simulink model "Wall_Model_Version_1_8_2016a"  (R2016a)
settings: Solver=ode3  StartTime=0.0  StopTime=inf  FixedStep=Ts  RelTol=1e-3
InitFcn:
  | clc;
  | clear all;
  | close all;
  | addpath('D:\Aravind_A0164966M_EE5003\Matlab files\3r2c model')
  | Ts=1
  | Duration=36000;
  | %% Coefficients of Rs and Cs
  | 
  | %% Front Wall
  | l1 = 7.37;
  | b1 = 2.63;
  | y1 = 0.5;
  | x1 = 0.33;
  | y2 = 0.5;
  | x2 = 0.33;
  | x3 = 0.33;
  | 
  | %% Left Wall
  | l2 = 10.11;
  | b2 = 2.63;
  | y3 = 0.5;
  | x4 = 0.33;
  | y4 = 0.5;
  | x5 = 0.33;
  | x6 = 0.33;
  | 
  | %% Left Wall Glass
  | x4_g = 0.5;
  | x5_g = 0.5;
  | y3_g = 1;
  | 
  | %% Right Wall
  | l3 = 7.37;
  | b3 = 2.63;
  | y5 = 0.5;
  | x7 = 0.33;
  | y6 = 0.5;
  | x8 = 0.33;
  | x9 = 0.33;
  | 
  | %% Back Wall
  | l4 = 10.11;
  | b4 = 2.63;
  | y7 = 1;
  | x10 = 0.5;
  | %y8 = 0.5;
  | x11 = 0.5;
  | %x12= 0.33;
  | 
  | %% Roof
  | l5 = 10.11;
  | b5 = 7.37;
  | y9 = 0.5;
  | x13 = 0.33;
  | y10 = 0.5;
  | x14 = 0.33;
  | x15 = 0.33;
  | 
  | %% Floor
  | l6 = 10.11;
  | b6 = 7.37;
  | y11 = 0.5;
  | x16 = 0.33;
  | y12 = 0.5;
  | x17 = 0.33;
  | x18 = 0.33;
  | 
  | %%Areas
  | A1 = l1 * b1;
  | A2 = l2 * b2;
  | A3 = l3 * b3;
  | A4 = l4 * b4;
  | A5 = l5 * b5;
  | A6 = l6 * b6;
  | 
  | %% Initial Temperatures at the surfaces
  | T1_initial_front=301;
  | T2_initial_front=300;
  | 
  | T1_initial_left=301;
  | T2_initial_left=300;
  | 
  | T1_initial_right=301;
  | T2_initial_right=300;
  | 
  | T1_initial_back=301;
  | T2_initial_back=300;
  | 
  | T1_initial_roof=301;
  | T2_initial_roof=300;
  | 
  | T1_initial_floor=301;
  | T2_initial_floor=300;
  | 
  | %ri = 0.1300; % m2 K/W resistance of inner surface of brick wall
  | %rso = 0.04; % m2 K/W resistance of outer surface of the wall
  | 
  | ri = 0;
  | rso = 0;
  | %% Density of Building materials in the room
  | p_conc    = 2400; % kg/m3 density of concrete
  | p_pstr     = 850; % kg/m3 density of plastering
  | p_gb       = 1100; % kg/m3 density of gypsum board
  | p_glass    = 2530; % kg/m3 density of glass
  | p_swood  = 550;   % kg/m3 density of soft-wood
  | 
  | %% Thermal heat capacity of the building materials in the room
  | c_conc    = 840;  % J/kg K heat capacity of concrete
  | c_pstr     = 1000;  %J/kg K heat capacity of plastering
  | c_gb       = 700; % J/kg K heat capacity of gypsum board
  | c_glass    = 840;  % J/kg K heat capacity of glass
  | c_swood  = 1700; % J/kg K heat capacity of soft-wood
  | 
  | %% Thermal conductivity(lamda) of building materials in the room
  | l_conc    = 0.8;  % W/m K Thermal conductivity of concrete
  | l_pstr     = 0.013;  % W/m K Thermal conductivity of plastering
  | l_gb       = 0.35; % W/m K Thermal conductivity of gypsum board
  | l_glass    = 0.8;  % W/m K Thermal conductivity of glass
  | l_swood  = 0.08; % W/m K Thermal conductivity of soft-wood
  | 
  | %% Standard thickness of materials used
  | d_conc = 0.01;  % m Thickness of concrete BCA standard
  | d_pstr = 0.005; % m Thickness of plastering BCA standard
  | d_glass = 0.015; % m Thickness of glass wall widely used
  | d_swood = 0.01; % m Thickness of softwood on the right wall
  | d_gb = 0.015; % m Thickness of gypsum board
  | 
  | %% Resistance and Capacitance of front Wall
  | Rth1 =( ri + rso + (d_conc/l_conc) + (d_pstr/l_pstr))/(A1); % Thermal resistance
  | Cth1 = A1*(d_conc*p_conc*c_conc + d_pstr*p_pstr*c_pstr) ; % Thermal Capacitance
  | 
  | %% Resistance and Capacitance of left Wall concrete
  | A_conc = A2 * 0.5; % Half of the wall on the left is  glass wall
  | Rth2 =( ri + rso + (d_conc/l_conc) + (d_pstr/l_pstr))/(A_conc); % Thermal resistance
  | Cth2 = A_conc*(d_conc*p_conc*c_conc + d_pstr*p_pstr*c_pstr); % Thermal Capacitance
  | 
  | %% Resistance and Capacitance of left Wall glass
  | A_glass = A2 * 0.5; % Half of the wall on the left is  glass wall
  | Rth2_g =(d_glass/l_glass) /(A_glass); % Thermal resistance
  | Cth2_g = A_glass*(d_glass*p_glass*c_glass ); % Thermal Capacitance
  | 
  | %% Resistance and Capacitance of right Wall
  | Rth3 = ( ri + rso+ (d_conc/l_conc) + (d_swood/l_swood))/(A3);% Thermal resistance
  | Cth3 = A3*(d_swood*p_swood*c_swood + d_conc*p_conc*c_conc ); % Thermal Capacitance
  | 
  | %% Resistance and Capacitance of back Wall
  | Rth4 =(d_glass/l_glass) /(A4); % Thermal resistance
  | Cth4 = A4*(d_glass*p_glass*c_glass ); % Thermal Capacitance
  | 
  | %% Resistance and Capacitance of roof Wall
  | Rth5 = (d_gb/l_gb)/(A5);% Thermal resistance
  | Cth5 = A5*(d_gb*p_gb*c_gb ); % Thermal Capacitance
  | 
  | %% Resistance and Capacitance of floor Wall
  | Rth6 = (d_gb/l_gb)/(A6);% Thermal resistance
  | Cth6 = A6*(d_gb*p_gb*c_gb ); % Thermal Capacitance
  | 
  | %% Volume and mass of room
  | density_of_air = 1.184; % kg/m3 at 25 deg. K
  | volume = l1*l2*b1; % m3
  | mass = volume * density_of_air ;% kg
  | specific_heat = 1.005; % J/kg deg.K
  | tic;
libraries: powerlib x70, simulink x1
settings Model: Creator=elekkr  LastModifiedBy=e0154145
settings DataIOCC: LimitDataPoints=on  SaveFormat=Array
settings DebuggingCC: UnconnectedInputMsg=none  UnconnectedOutputMsg=none  UnconnectedLineMsg=none
settings HardwareCC: ProdBitPerPointer=32  ProdLargestAtomicFloat=None  ProdIntDivRoundTo=Undefined  ProdEndianess=Unspecified  ProdWordSize=32  ProdHWDeviceType=32-bit Generic
settings ModelReferenceCC: PropagateSignalLabelsOutOfModel=off
settings SimscapeCC: SimscapeNormalizeSystem=off

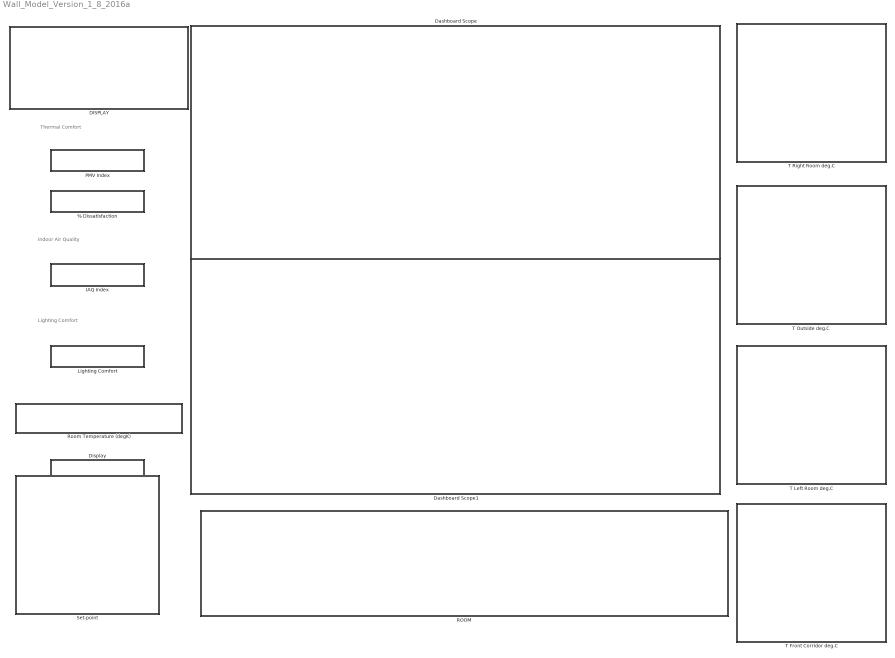
== system Wall_Model_Version_1_8_2016a ==
  note: Thermal Comfort
  note: Indoor Air Quality
  note: Lighting Comfort
  % Dissatisfaction : Subsystem  Description=Replaced Block  mask(Replaced Block){}
      mask help: This block has been replaced with an empty subsystem because it used functionality that is unavailable in Simulink R2016a.
      mask Display: fprintf('Replaced: %s\n','Dashboard Widget')
  DISPLAY : Subsystem  mask(GBIC - Simulation Speed){}
      settings: AttributesFormatString=141.41
      mask Display: fprintf('Simulation_Time_Elapsed=3536.00 seconds\nPhysical_Time_Elapsed=70.38 seconds\nSimulation_Speed=50.24 times')
  Dashboard Scope : Subsystem  DialogController=hmiCreateDDGDialog  IsWebBlock=on  mask(MWDashboardBlock){webBlockId=3fff6f15-1f4d-4564-ab32-a1e668a3884d, webBlockType=sdiscope, ShowInitialText=on, HMISrcModelName=Wall_Model_Version_1_8_2016a}
      mask prompts: webBlockId "WebBlock Id"; webBlockType "WebBlock Type"; HMISrcModelName "Source Model"
      mask help: SimulinkHMI:dialogs:HMIScopeDialogDesc
      mask Help: helpview([docroot '/mapfiles/simulink.map'], 'hmi_scope')
      mask Display:
      | if strcmp(get_param(bdroot(gcb),'BlockDiagramType'), 'library')
      |     image([(matlabroot) '/toolbox/simulink/hmi/icons/DashboardScope.png']);
      | end
  Dashboard Scope1 : Subsystem  DialogController=hmiCreateDDGDialog  IsWebBlock=on  mask(MWDashboardBlock){webBlockId=a7778c0b-7014-479c-88b7-c1742b1b2716, webBlockType=sdiscope, ShowInitialText=on, HMISrcModelName=Wall_Model_Version_1_8_2016a}
      mask prompts: webBlockId "WebBlock Id"; webBlockType "WebBlock Type"; HMISrcModelName "Source Model"
      mask help: SimulinkHMI:dialogs:HMIScopeDialogDesc
      mask Help: helpview([docroot '/mapfiles/simulink.map'], 'hmi_scope')
      mask Display:
      | if strcmp(get_param(bdroot(gcb),'BlockDiagramType'), 'library')
      |     image([(matlabroot) '/toolbox/simulink/hmi/icons/DashboardScope.png']);
      | end
  Display : Subsystem  Description=Replaced Block  mask(Replaced Block){}
      mask help: This block has been replaced with an empty subsystem because it used functionality that is unavailable in Simulink R2016a.
      mask Display: fprintf('Replaced: %s\n','Dashboard Widget')
  IAQ Index : Subsystem  Description=Replaced Block  mask(Replaced Block){}
      mask help: This block has been replaced with an empty subsystem because it used functionality that is unavailable in Simulink R2016a.
      mask Display: fprintf('Replaced: %s\n','Dashboard Widget')
  Lighting Comfort : Subsystem  Description=Replaced Block  mask(Replaced Block){}
      mask help: This block has been replaced with an empty subsystem because it used functionality that is unavailable in Simulink R2016a.
      mask Display: fprintf('Replaced: %s\n','Dashboard Widget')
  PMV Index : Subsystem  Description=Replaced Block  mask(Replaced Block){}
      mask help: This block has been replaced with an empty subsystem because it used functionality that is unavailable in Simulink R2016a.
      mask Display: fprintf('Replaced: %s\n','Dashboard Widget')
  ROOM : Subsystem
  Room Temperature (degK) : Subsystem  DialogController=hmiCreateDDGDialog  IsWebBlock=on  mask(MWDashboardBlock){webBlockId=20cf081a-ecf9-409a-b722-1806c1b228f7, webBlockType=lineargauge, ShowInLibBrowser=on, ShowInitialText=on, HMISrcModelName=Wall_Model_Version_1_8_2016a}
      mask prompts: webBlockId "WebBlock Id"; webBlockType "WebBlock Type"; HMISrcModelName "Source Model"
      mask help: SimulinkHMI:dialogs:LinearGaugeDialogDesc
      mask Help: helpview([docroot '/mapfiles/simulink.map'], 'hmi_linear_gauge')
      mask Display:
      | if strcmp(get_param(bdroot(gcb),'BlockDiagramType'), 'library')
      |     image([(matlabroot) '/toolbox/simulink/hmi/icons/LinearGauge.png']);
      | end
  Set-point : Subsystem  DialogController=hmiCreateDDGDialog  IsWebBlock=on  mask(MWDashboardBlock){webBlockId=ec28f16f-92e5-498c-80e5-da4bfa106054, webBlockType=discreteknob, ShowInLibBrowser=on, ShowInitialText=on, HMISrcModelName=Wall_Model_Version_1_8_2016a}
      mask prompts: webBlockId "WebBlock Id"; webBlockType "WebBlock Type"; HMISrcModelName "Source Model"
      mask help: Set value to tune parameters or variables.
      mask Help: helpview([docroot '/mapfiles/simulink.map'], 'hmi_rotary_switch')
      mask Display:
      | if strcmp(get_param(bdroot(gcb),'BlockDiagramType'),'library')
      |  image([(matlabroot) '/toolbox/simulink/hmi/icons/DiscreteKnob.png'])
      | end
  T Front Corridor deg.C : Subsystem  DialogController=hmiCreateDDGDialog  IsWebBlock=on  mask(MWDashboardBlock){webBlockId=cdae9e03-d357-446c-8d97-860cc5abe23b, webBlockType=discreteknob, ShowInLibBrowser=on, ShowInitialText=on, HMISrcModelName=Wall_Model_Version_1_8_2016a}
      mask prompts: webBlockId "WebBlock Id"; webBlockType "WebBlock Type"; HMISrcModelName "Source Model"
      mask help: Set value to tune parameters or variables.
      mask Help: helpview([docroot '/mapfiles/simulink.map'], 'hmi_rotary_switch')
      mask Display:
      | if strcmp(get_param(bdroot(gcb),'BlockDiagramType'),'library')
      |  image([(matlabroot) '/toolbox/simulink/hmi/icons/DiscreteKnob.png'])
      | end
  T Left Room deg.C : Subsystem  DialogController=hmiCreateDDGDialog  IsWebBlock=on  mask(MWDashboardBlock){webBlockId=223c3754-b648-4b30-8efa-3705ba18b69c, webBlockType=discreteknob, ShowInLibBrowser=on, ShowInitialText=on, HMISrcModelName=Wall_Model_Version_1_8_2016a}
      mask prompts: webBlockId "WebBlock Id"; webBlockType "WebBlock Type"; HMISrcModelName "Source Model"
      mask help: Set value to tune parameters or variables.
      mask Help: helpview([docroot '/mapfiles/simulink.map'], 'hmi_rotary_switch')
      mask Display:
      | if strcmp(get_param(bdroot(gcb),'BlockDiagramType'),'library')
      |  image([(matlabroot) '/toolbox/simulink/hmi/icons/DiscreteKnob.png'])
      | end
  T Outside deg.C : Subsystem  DialogController=hmiCreateDDGDialog  IsWebBlock=on  mask(MWDashboardBlock){webBlockId=3d2b147f-38bc-43af-8396-33a98fe59ecc, webBlockType=discreteknob, ShowInLibBrowser=on, ShowInitialText=on, HMISrcModelName=Wall_Model_Version_1_8_2016a}
      mask prompts: webBlockId "WebBlock Id"; webBlockType "WebBlock Type"; HMISrcModelName "Source Model"
      mask help: Set value to tune parameters or variables.
      mask Help: helpview([docroot '/mapfiles/simulink.map'], 'hmi_rotary_switch')
      mask Display:
      | if strcmp(get_param(bdroot(gcb),'BlockDiagramType'),'library')
      |  image([(matlabroot) '/toolbox/simulink/hmi/icons/DiscreteKnob.png'])
      | end
  T Right Room deg.C : Subsystem  DialogController=hmiCreateDDGDialog  IsWebBlock=on  mask(MWDashboardBlock){webBlockId=eb2fffaf-f8f3-43a1-940d-0b33cab81fdd, webBlockType=discreteknob, ShowInLibBrowser=on, ShowInitialText=on, HMISrcModelName=Wall_Model_Version_1_8_2016a}
      mask prompts: webBlockId "WebBlock Id"; webBlockType "WebBlock Type"; HMISrcModelName "Source Model"
      mask help: Set value to tune parameters or variables.
      mask Help: helpview([docroot '/mapfiles/simulink.map'], 'hmi_rotary_switch')
      mask Display:
      | if strcmp(get_param(bdroot(gcb),'BlockDiagramType'),'library')
      |  image([(matlabroot) '/toolbox/simulink/hmi/icons/DiscreteKnob.png'])
      | end

== system Wall_Model_Version_1_8_2016a/% Dissatisfaction ==

== system Wall_Model_Version_1_8_2016a/DISPLAY ==
  Disp_Function : M-S-Function  FunctionName=fn_Display

== system Wall_Model_Version_1_8_2016a/Dashboard Scope ==

== system Wall_Model_Version_1_8_2016a/Dashboard Scope1 ==

== system Wall_Model_Version_1_8_2016a/Display ==

== system Wall_Model_Version_1_8_2016a/IAQ Index ==

== system Wall_Model_Version_1_8_2016a/Lighting Comfort ==

== system Wall_Model_Version_1_8_2016a/PMV Index ==

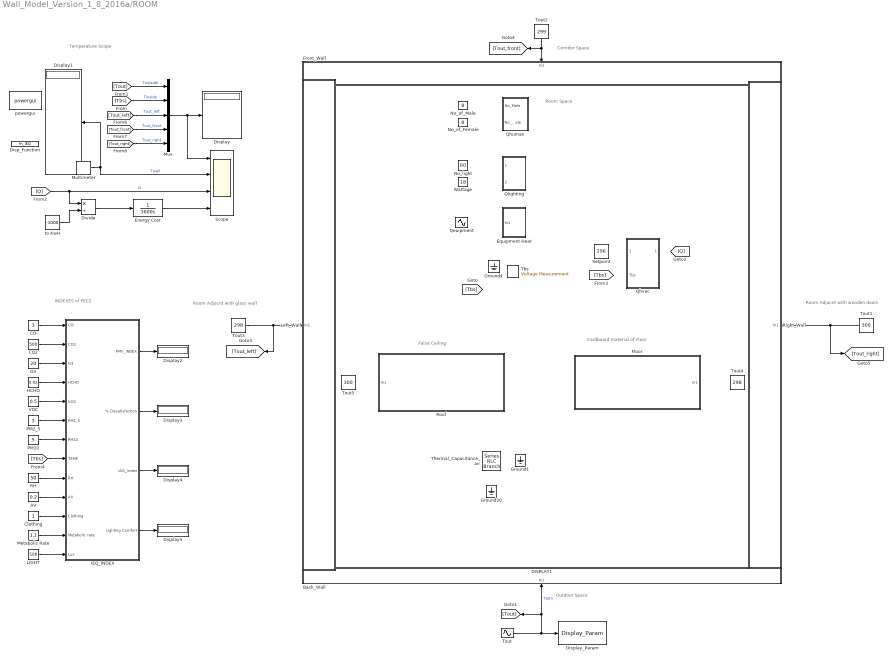
== system Wall_Model_Version_1_8_2016a/ROOM ==
  note: INDEXES of FEC2
  note: False Ceiling
  note: Cardboard material of Floor
  note: Room Adjacnt with wooden doors
  note: Corridor Space
  note: Room Adjacnt with glass wall
  note: Outdoor Space
  note: Room Space
  note: Temperature Scope
  AV : Constant  Value=0.2
  Back_Wall : Subsystem
      mask Display: fprintf('Temperature Outside= 303 deg. K\n')
  CO : Constant  Value=3
  CO2 : Constant  Value=500
  Clothing : Constant
  DISPLAY1 : Subsystem  mask(GBIC - Simulation Speed){}
      settings: AttributesFormatString=35.01
  Disp_Function : M-S-Function  FunctionName=fn_IEQ
  Display{,1..5} (6 alike) : Display
  Display_Param : M-S-Function  FunctionName=Display_Param
  Divide : Product  Inputs=*/
  Energy Cost : TransferFcn  Denominator=[3600 0]
  Equipment Heat : Subsystem
  Floor : Subsystem
      mask Display: fprintf('Temperature \n Below= \n298 deg. K\n')
  Front_Wall : Subsystem
      mask Display: fprintf('Temperature Corridor= 299 deg. K\n')
  Ground1 : powerlib/Elements/Ground  LConnTagsString=a
  Ground20 : powerlib/Elements/Ground  LConnTagsString=a
  Ground4 : powerlib/Elements/Ground  LConnTagsString=a
  HCHO : Constant  Value=0.02
  IEQ_INDEX : Subsystem
  LIGHT : Constant  Value=500
  Left_Wall : Subsystem
      mask Display: fprintf('Temperature \n Left Room= \n298 deg. K\n')
  Metabolic Rate : Constant  Value=1.1
  Multimeter : powerlib/Measurements/Multimeter  PhasorSimulation=off  OutputType=Complex  sel=1  L=12  Gain=0  yselected={}  PSBOutputType=1  PSBequivalent=0  AxesSetting=[0,0.1,-100,100]  Display=0  SavedBlockNames=-11
  Mux : Mux  Inputs=5
  No_light : Constant  Value=60
  No_of_Female : Constant  Value=8
  No_of_Male : Constant  Value=8
  O3 : Constant  Value=20
  PM10 : Constant  Value=5
  PM2_5 : Constant  Value=3
  Qeuipment : Sin  Amplitude=200  Bias=3200  Frequency=2*pi/(12*3600)  SampleTime=0
  Qhuman : Subsystem
  Qhvac : Subsystem
  Qlighting : Subsystem
  RH : Constant  Value=50
  Right_Wall : Subsystem
      mask Display: fprintf('Temperature \n Right Room= \n300 deg. K\n')
  Roof : Subsystem
      mask Display: fprintf('Temperature \n Above Roof= \n300 deg. K\n')
  Scope : Scope  NumInputPorts=4
  Setpoint : Constant  Value=296
  Tbs : powerlib/Measurements/Voltage Measurement  PhasorSimulation=off  OutputType=Magnitude  PSBequivalent=0
  Thermal_Capacitance_air : powerlib/Elements/Series RLC Branch  LConnTagsString=__new0  RConnTagsString=__new0  BranchType=C  Resistance=0  Inductance=1e-3  SetiL0=off  InitialCurrent=0  Capacitance=density_of_air * volume * specific_heat  Setx0=on  InitialVoltage=298  Measurements=Branch voltage
  Tout : Sin  Amplitude=0  Bias=303  Frequency=2*pi/(12*3600)  SampleTime=0
  Tout1 : Constant  Value=300
  Tout2 : Constant  Value=299
  Tout3 : Constant  Value=298
  Tout4 : Constant  Value=298
  Tout5 : Constant  Value=300
  VOC : Constant  Value=0.5
  Wattage : Constant  Value=18
  powergui : powerlib/powergui  Priority=1  SimulationMode=Discrete  SampleTime=Ts  frequency=60  Iterations=50  frequencyindice=0  Pbase=100e6  ErrMax=1e-4  UnitsV=kV  UnitsW=MW  buscounter=0  FunctionMessages=off  echomessages=off  EnableUseOfTLC=off  CurrentSourceSwitches=off  DisableSnubberDevices=off  DisableRonSwitches=off  DisableVfSwitches=off  DisplayEquations=off  SolverType=Tustin/Backward Euler (TBE)  Interpol=off  ExternalGateDelay=off  methode=off  Ts=100  x0status=blocks  SPID=off  SwTol=0  HookPort=off  RestoreLinks=warning  ResistiveCurrentMeasurement=off  Frange=[0:2:500]  Ylog=off  Xlog=on  ShowGrid=off  save=off  variable=ZData  structure=0  ZoomFFT=off  StartTime=0.0  cycles=1  DisplayStyle=1  fundamental=60  FreqAxis=off  MaxFrequency=1000  frequencyindicesteady=1  RmsSteady=1  display=off
  to KwH : Constant  Value=-1000
  wires:
  No_of_Female/1 -> Qhuman/2(No_Female)
  Tout5/1 -> Roof/1(In1)
  [Tbs] -> Qhvac/2(Tbs)
  Tout3/1 -> [Tout_left], Left_Wall/1(In1)
  [Tout] -> Mux/1  "Toutside"
  [Q] -> Scope/3, Divide/1  "Q"
  Setpoint/1 -> Qhvac/1(Setpoint)
  Qhvac/1(Qhvac) -> [Q]
  Tout1/1 -> [Tout_right], Right_Wall/1(In1)
  Tbs/1 -> [Tbs]
  Tout/1 -> Display_Param/1, Back_Wall/1(In1), [Tout]  "Tatm"
  Tout4/1 -> Floor/1(In1)
  [Tout_front] -> Mux/4  "Tout_front"
  No_light/1 -> Qlighting/1("No_light ")
  Tout2/1 -> [Tout_front], Front_Wall/1(In1)
  Multimeter/1 -> Scope/2, Display1/1  "Twall"
  [Tout_right] -> Mux/5  "Tout_right"
  [Tout_left] -> Mux/3  "Tout_left"
  No_of_Male/1 -> Qhuman/1("No_Male ")
  Wattage/1 -> Qlighting/2(Wattage)
  Mux/1 -> Scope/1, Display/1
  Qeuipment/1 -> Equipment Heat/1(In1)
  [Tbs] -> Mux/2  "Tinside"
  to KwH/1 -> Divide/2
  Energy Cost/1 -> Scope/4
  Divide/1 -> Energy Cost/1
  [Tbs] -> IEQ_INDEX/8(TEMP)
  CO/1 -> IEQ_INDEX/1(CO)
  PM10/1 -> IEQ_INDEX/7(PM10)
  PM2_5/1 -> IEQ_INDEX/6(PM2_5)
  VOC/1 -> IEQ_INDEX/5(VOC)
  HCHO/1 -> IEQ_INDEX/4(HCHO)
  O3/1 -> IEQ_INDEX/3(O3)
  CO2/1 -> IEQ_INDEX/2(CO2)
  RH/1 -> IEQ_INDEX/9(RH)
  AV/1 -> IEQ_INDEX/10(AV)
  Clothing/1 -> IEQ_INDEX/11(Clothing)
  IEQ_INDEX/1(PMV_INDEX) -> Display2/1
  IEQ_INDEX/2("% Dissatisfaction ") -> Display3/1
  LIGHT/1 -> IEQ_INDEX/13(Lux)
  Metabolic Rate/1 -> IEQ_INDEX/12(Metabolic rate)
  IEQ_INDEX/3(IAQ_Index) -> Display4/1
  IEQ_INDEX/4(Lighting Comfort) -> Display5/1
  connections:
  Ground4/LConn1 -- Tbs/LConn2
  Equipment Heat/RConn1 -- Qhvac/RConn1 -- Right_Wall/RConn1 -- Back_Wall/RConn1 -- Floor/RConn1 -- Roof/RConn1 -- Left_Wall/RConn1 -- Tbs/LConn1 -- Qlighting/RConn1 -- Qhuman/RConn1 -- Front_Wall/RConn1
  Ground20/LConn1 -- Thermal_Capacitance_air/RConn1
  Thermal_Capacitance_air/LConn1 -- Ground1/LConn1

== system Wall_Model_Version_1_8_2016a/Room Temperature (degK) ==

== system Wall_Model_Version_1_8_2016a/Set-point ==

== system Wall_Model_Version_1_8_2016a/T Front Corridor deg.C ==

== system Wall_Model_Version_1_8_2016a/T Left Room deg.C ==

== system Wall_Model_Version_1_8_2016a/T Outside deg.C ==

== system Wall_Model_Version_1_8_2016a/T Right Room deg.C ==

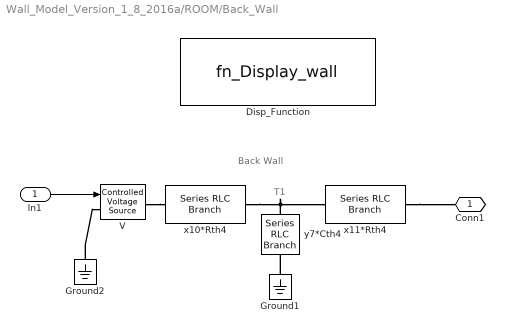
== system Wall_Model_Version_1_8_2016a/ROOM/Back_Wall ==
  note: T1
  note: Back Wall
  In1 : Inport
  Disp_Function : M-S-Function  FunctionName=fn_Display_wall
  Ground1 : powerlib/Elements/Ground  LConnTagsString=a
  Ground2 : powerlib/Elements/Ground  LConnTagsString=a
  V : powerlib/Electrical Sources/Controlled Voltage Source  Initialize=on  Source_Type=AC  Amplitude=0  Phase=0  Frequency=0  Measurements=None
  x10*Rth4 : powerlib/Elements/Series RLC Branch  LConnTagsString=__new0  RConnTagsString=__new0  BranchType=R  Resistance=x10*Rth4  Inductance=1e-3  SetiL0=off  InitialCurrent=0  Capacitance=1e-6  Setx0=off  InitialVoltage=0  Measurements=None
  x11*Rth4 : powerlib/Elements/Series RLC Branch  LConnTagsString=__new0  RConnTagsString=__new0  BranchType=R  Resistance=x11*Rth4  Inductance=1e-3  SetiL0=off  InitialCurrent=0  Capacitance=1e-6  Setx0=off  InitialVoltage=0  Measurements=None
  y7*Cth4 : powerlib/Elements/Series RLC Branch  LConnTagsString=__new0  RConnTagsString=__new0  BranchType=C  Resistance=0  Inductance=1e-3  SetiL0=off  InitialCurrent=0  Capacitance=y7*Cth4  Setx0=on  InitialVoltage=T1_initial_back  Measurements=Branch voltage
  Conn1 : PMIOPort  Side=Right
  wires:
  In1/1 -> V/1
  connections:
  Ground2/LConn1 -- V/LConn1
  V/RConn1 -- x10*Rth4/LConn1
  x10*Rth4/RConn1 -- y7*Cth4/LConn1 -- x11*Rth4/LConn1
  Ground1/LConn1 -- y7*Cth4/RConn1
  x11*Rth4/RConn1 -- Conn1/RConn1

== system Wall_Model_Version_1_8_2016a/ROOM/DISPLAY1 ==
  Disp_Function : M-S-Function  FunctionName=fn_Display_Room

== system Wall_Model_Version_1_8_2016a/ROOM/Equipment Heat ==
  In1 : Inport
  Ground20 : powerlib/Elements/Ground  LConnTagsString=a
  I1 : powerlib/Electrical Sources/Controlled Current Source  Initialize=off  Source_Type=AC  Amplitude=1  Phase=0  Frequency=0  Measurements=None
  Conn1 : PMIOPort  Side=Right
  wires:
  In1/1 -> I1/1
  connections:
  Ground20/LConn1 -- I1/LConn1
  I1/RConn1 -- Conn1/RConn1

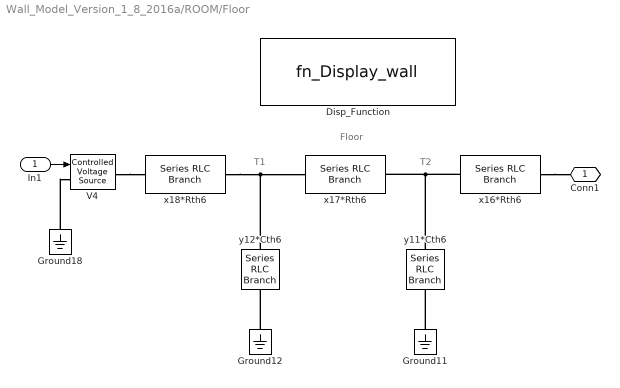
== system Wall_Model_Version_1_8_2016a/ROOM/Floor ==
  note: T2
  note: T1
  note: Floor
  In1 : Inport
  Disp_Function : M-S-Function  FunctionName=fn_Display_wall
  Ground11 : powerlib/Elements/Ground  LConnTagsString=a
  Ground12 : powerlib/Elements/Ground  LConnTagsString=a
  Ground18 : powerlib/Elements/Ground  LConnTagsString=a
  V4 : powerlib/Electrical Sources/Controlled Voltage Source  Initialize=on  Source_Type=AC  Amplitude=0  Phase=0  Frequency=0  Measurements=None
  x16*Rth6 : powerlib/Elements/Series RLC Branch  LConnTagsString=__new0  RConnTagsString=__new0  BranchType=R  Resistance=x16*Rth6  Inductance=1e-3  SetiL0=off  InitialCurrent=0  Capacitance=1e-6  Setx0=off  InitialVoltage=0  Measurements=None
  x17*Rth6 : powerlib/Elements/Series RLC Branch  LConnTagsString=__new0  RConnTagsString=__new0  BranchType=R  Resistance=x17*Rth6  Inductance=1e-3  SetiL0=off  InitialCurrent=0  Capacitance=1e-6  Setx0=off  InitialVoltage=0  Measurements=None
  x18*Rth6 : powerlib/Elements/Series RLC Branch  LConnTagsString=__new0  RConnTagsString=__new0  BranchType=R  Resistance=x18*Rth6  Inductance=1e-3  SetiL0=off  InitialCurrent=0  Capacitance=1e-6  Setx0=off  InitialVoltage=0  Measurements=None
  y11*Cth6 : powerlib/Elements/Series RLC Branch  LConnTagsString=__new0  RConnTagsString=__new0  BranchType=C  Resistance=0  Inductance=1e-3  SetiL0=off  InitialCurrent=0  Capacitance=y11*Cth6  Setx0=on  InitialVoltage=T1_initial_floor  Measurements=Branch voltage
  y12*Cth6 : powerlib/Elements/Series RLC Branch  LConnTagsString=__new0  RConnTagsString=__new0  BranchType=C  Resistance=0  Inductance=1e-3  SetiL0=off  InitialCurrent=0  Capacitance=y12*Cth6  Setx0=on  InitialVoltage=T2_initial_floor  Measurements=Branch voltage
  Conn1 : PMIOPort  Side=Right
  wires:
  In1/1 -> V4/1
  connections:
  V4/RConn1 -- x18*Rth6/LConn1
  y11*Cth6/LConn1 -- x16*Rth6/LConn1 -- x17*Rth6/RConn1
  y12*Cth6/LConn1 -- x18*Rth6/RConn1 -- x17*Rth6/LConn1
  Ground18/LConn1 -- V4/LConn1
  Ground11/LConn1 -- y11*Cth6/RConn1
  Ground12/LConn1 -- y12*Cth6/RConn1
  x16*Rth6/RConn1 -- Conn1/RConn1

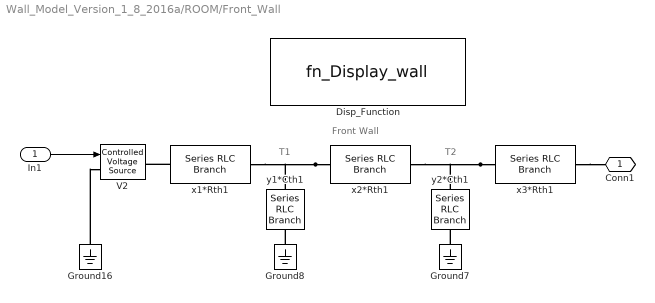
== system Wall_Model_Version_1_8_2016a/ROOM/Front_Wall ==
  note: Front Wall
  note: T2
  note: T1
  In1 : Inport
  Disp_Function : M-S-Function  FunctionName=fn_Display_wall
  Ground16 : powerlib/Elements/Ground  LConnTagsString=a
  Ground7 : powerlib/Elements/Ground  LConnTagsString=a
  Ground8 : powerlib/Elements/Ground  LConnTagsString=a
  V2 : powerlib/Electrical Sources/Controlled Voltage Source  Initialize=on  Source_Type=AC  Amplitude=0  Phase=0  Frequency=0  Measurements=None
  x1*Rth1 : powerlib/Elements/Series RLC Branch  LConnTagsString=__new0  RConnTagsString=__new0  BranchType=R  Resistance=x1*Rth1  Inductance=1e-3  SetiL0=off  InitialCurrent=0  Capacitance=1e-6  Setx0=off  InitialVoltage=0  Measurements=None
  x2*Rth1 : powerlib/Elements/Series RLC Branch  LConnTagsString=__new0  RConnTagsString=__new0  BranchType=R  Resistance=x2*Rth1  Inductance=1e-3  SetiL0=off  InitialCurrent=0  Capacitance=1e-6  Setx0=off  InitialVoltage=0  Measurements=None
  x3*Rth1 : powerlib/Elements/Series RLC Branch  LConnTagsString=__new0  RConnTagsString=__new0  BranchType=R  Resistance=x3*Rth1  Inductance=1e-3  SetiL0=off  InitialCurrent=0  Capacitance=1e-6  Setx0=off  InitialVoltage=0  Measurements=None
  y1*Cth1 : powerlib/Elements/Series RLC Branch  LConnTagsString=__new0  RConnTagsString=__new0  BranchType=C  Resistance=0  Inductance=1e-3  SetiL0=off  InitialCurrent=0  Capacitance=y1*Cth1  Setx0=on  InitialVoltage=T1_initial_front  Measurements=Branch voltage
  y2*Cth1 : powerlib/Elements/Series RLC Branch  LConnTagsString=__new0  RConnTagsString=__new0  BranchType=C  Resistance=0  Inductance=1e-3  SetiL0=off  InitialCurrent=0  Capacitance=y2*Cth1  Setx0=on  InitialVoltage=T2_initial_front  Measurements=Branch voltage
  Conn1 : PMIOPort  Side=Right
  wires:
  In1/1 -> V2/1
  connections:
  Ground7/LConn1 -- y2*Cth1/RConn1
  x2*Rth1/LConn1 -- x1*Rth1/RConn1 -- y1*Cth1/LConn1
  x3*Rth1/LConn1 -- x2*Rth1/RConn1 -- y2*Cth1/LConn1
  Ground16/LConn1 -- V2/LConn1
  Ground8/LConn1 -- y1*Cth1/RConn1
  x1*Rth1/LConn1 -- V2/RConn1
  x3*Rth1/RConn1 -- Conn1/RConn1

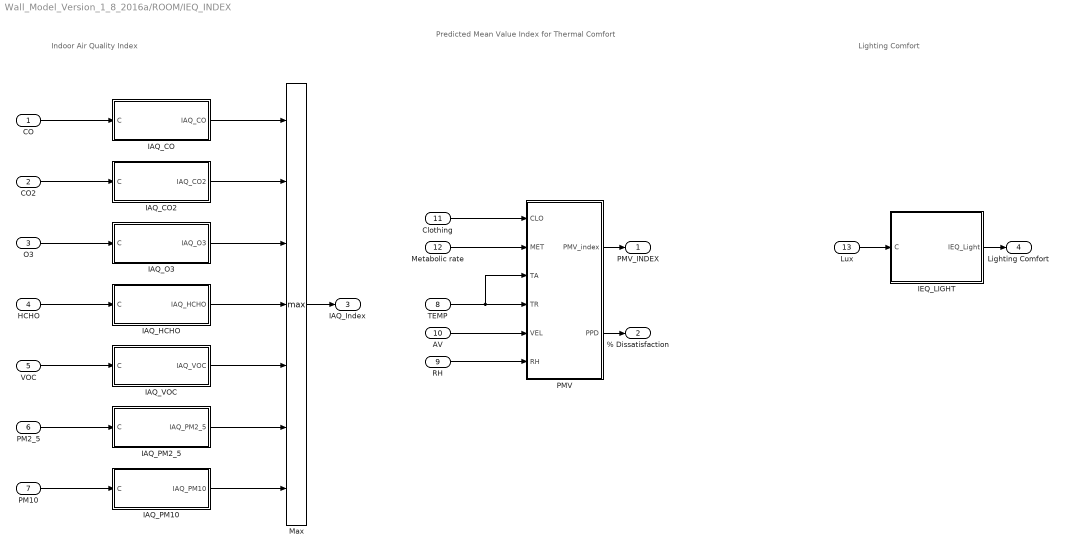
== system Wall_Model_Version_1_8_2016a/ROOM/IEQ_INDEX ==
  note: Indoor Air Quality Index
  note: Predicted Mean Value Index
      | for Thermal Comfort
  note: Lighting Comfort
  CO : Inport
  CO2 : Inport  Port=2
  O3 : Inport  Port=3
  HCHO : Inport  Port=4
  VOC : Inport  Port=5
  PM2_5 : Inport  Port=6
  PM10 : Inport  Port=7
  TEMP : Inport  Port=8
  RH : Inport  Port=9
  AV : Inport  Port=10
  Clothing : Inport  Port=11
  Metabolic rate : Inport  Port=12
  Lux : Inport  Port=13
  IAQ_CO : MATLAB Function  TreatAsAtomicUnit=on
  IAQ_CO2 : MATLAB Function  TreatAsAtomicUnit=on
  IAQ_HCHO : MATLAB Function  TreatAsAtomicUnit=on
  IAQ_O3 : MATLAB Function  TreatAsAtomicUnit=on
  IAQ_PM10 : MATLAB Function  TreatAsAtomicUnit=on
  IAQ_PM2_5 : MATLAB Function  TreatAsAtomicUnit=on
  IAQ_VOC : MATLAB Function  TreatAsAtomicUnit=on
  IEQ_LIGHT : MATLAB Function  TreatAsAtomicUnit=on
  Max : MinMax  Function=max  Inputs=7
  PMV : MATLAB Function  TreatAsAtomicUnit=on
  PMV_INDEX : Outport
  "% Dissatisfaction " : Outport  Port=2
  IAQ_Index : Outport  Port=3
  Lighting Comfort : Outport  Port=4
  wires:
  CO/1 -> IAQ_CO/1(C)
  IAQ_PM10/1(IAQ_PM10) -> Max/7
  IAQ_VOC/1(IAQ_VOC) -> Max/5
  CO2/1 -> IAQ_CO2/1(C)
  PM2_5/1 -> IAQ_PM2_5/1(C)
  IAQ_CO/1(IAQ_CO) -> Max/1
  PM10/1 -> IAQ_PM10/1(C)
  IAQ_PM2_5/1(IAQ_PM2_5) -> Max/6
  IAQ_HCHO/1(IAQ_HCHO) -> Max/4
  IAQ_CO2/1(IAQ_CO2) -> Max/2
  HCHO/1 -> IAQ_HCHO/1(C)
  VOC/1 -> IAQ_VOC/1(C)
  IAQ_O3/1(IAQ_O3) -> Max/3
  O3/1 -> IAQ_O3/1(C)
  RH/1 -> PMV/6(RH)
  AV/1 -> PMV/5(VEL)
  TEMP/1 -> PMV/3(TA), PMV/4(TR)
  Metabolic rate/1 -> PMV/2(MET)
  Clothing/1 -> PMV/1(CLO)
  PMV/1(PMV_index) -> PMV_INDEX/1
  PMV/2(PPD) -> "% Dissatisfaction "/1
  Max/1 -> IAQ_Index/1
  Lux/1 -> IEQ_LIGHT/1(C)
  IEQ_LIGHT/1(IEQ_Light) -> Lighting Comfort/1

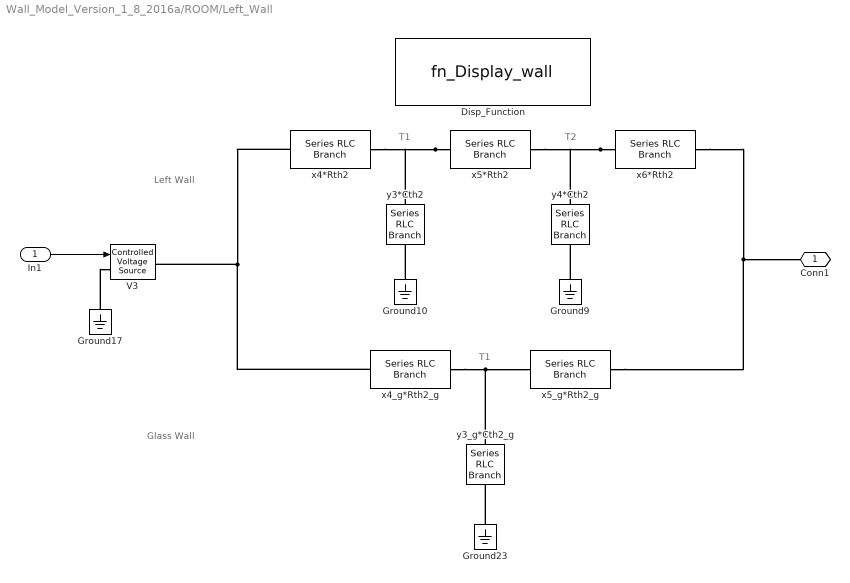
== system Wall_Model_Version_1_8_2016a/ROOM/Left_Wall ==
  note: T1
  note: Glass Wall
  note: Left Wall
  note: T2
  note: T1
  In1 : Inport
  Disp_Function : M-S-Function  FunctionName=fn_Display_wall
  Ground{9..10,17,23} (4 alike) : powerlib/Elements/Ground  LConnTagsString=a
  V3 : powerlib/Electrical Sources/Controlled Voltage Source  Initialize=on  Source_Type=AC  Amplitude=0  Phase=0  Frequency=0  Measurements=None
  x4*Rth2 : powerlib/Elements/Series RLC Branch  LConnTagsString=__new0  RConnTagsString=__new0  BranchType=R  Resistance=x4*Rth2  Inductance=1e-3  SetiL0=off  InitialCurrent=0  Capacitance=1e-6  Setx0=off  InitialVoltage=0  Measurements=None
  x4_g*Rth2_g : powerlib/Elements/Series RLC Branch  LConnTagsString=__new0  RConnTagsString=__new0  BranchType=R  Resistance=x4_g*Rth2_g  Inductance=1e-3  SetiL0=off  InitialCurrent=0  Capacitance=1e-6  Setx0=off  InitialVoltage=0  Measurements=None
  x5*Rth2 : powerlib/Elements/Series RLC Branch  LConnTagsString=__new0  RConnTagsString=__new0  BranchType=R  Resistance=x5*Rth2  Inductance=1e-3  SetiL0=off  InitialCurrent=0  Capacitance=1e-6  Setx0=off  InitialVoltage=0  Measurements=None
  x5_g*Rth2_g : powerlib/Elements/Series RLC Branch  LConnTagsString=__new0  RConnTagsString=__new0  BranchType=R  Resistance=x5_g*Rth2_g  Inductance=1e-3  SetiL0=off  InitialCurrent=0  Capacitance=1e-6  Setx0=off  InitialVoltage=0  Measurements=None
  x6*Rth2 : powerlib/Elements/Series RLC Branch  LConnTagsString=__new0  RConnTagsString=__new0  BranchType=R  Resistance=x6*Rth2  Inductance=1e-3  SetiL0=off  InitialCurrent=0  Capacitance=1e-6  Setx0=off  InitialVoltage=0  Measurements=None
  y3*Cth2 : powerlib/Elements/Series RLC Branch  LConnTagsString=__new0  RConnTagsString=__new0  BranchType=C  Resistance=0  Inductance=1e-3  SetiL0=off  InitialCurrent=0  Capacitance=y3*Cth2  Setx0=on  InitialVoltage=T1_initial_left  Measurements=Branch voltage
  y3_g*Cth2_g : powerlib/Elements/Series RLC Branch  LConnTagsString=__new0  RConnTagsString=__new0  BranchType=C  Resistance=0  Inductance=1e-3  SetiL0=off  InitialCurrent=0  Capacitance=y3_g*Cth2_g  Setx0=on  InitialVoltage=T1_initial_left  Measurements=Branch voltage
  y4*Cth2 : powerlib/Elements/Series RLC Branch  LConnTagsString=__new0  RConnTagsString=__new0  BranchType=C  Resistance=0  Inductance=1e-3  SetiL0=off  InitialCurrent=0  Capacitance=y4*Cth2  Setx0=on  InitialVoltage=T2_initial_left  Measurements=Branch voltage
  Conn1 : PMIOPort  Side=Right
  wires:
  In1/1 -> V3/1
  connections:
  x5*Rth2/LConn1 -- x4*Rth2/RConn1 -- y3*Cth2/LConn1
  x6*Rth2/LConn1 -- x5*Rth2/RConn1 -- y4*Cth2/LConn1
  x4*Rth2/LConn1 -- x4_g*Rth2_g/LConn1 -- V3/RConn1
  x6*Rth2/RConn1 -- x5_g*Rth2_g/RConn1 -- Conn1/RConn1
  Ground10/LConn1 -- y3*Cth2/RConn1
  y3_g*Cth2_g/LConn1 -- x4_g*Rth2_g/RConn1 -- x5_g*Rth2_g/LConn1
  Ground23/LConn1 -- y3_g*Cth2_g/RConn1
  Ground9/LConn1 -- y4*Cth2/RConn1
  Ground17/LConn1 -- V3/LConn1

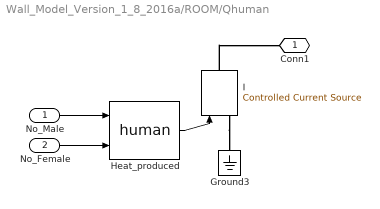
== system Wall_Model_Version_1_8_2016a/ROOM/Qhuman ==
  "No_Male " : Inport
  No_Female : Inport  Port=2
  Ground3 : powerlib/Elements/Ground  LConnTagsString=a
  Heat_produced : M-S-Function  FunctionName=human
  I : powerlib/Electrical Sources/Controlled Current Source  Initialize=on  Source_Type=AC  Amplitude=1  Phase=0  Frequency=0  Measurements=None
  Conn1 : PMIOPort  Side=Right
  wires:
  "No_Male "/1 -> Heat_produced/1
  Heat_produced/1 -> I/1
  No_Female/1 -> Heat_produced/2
  connections:
  I/LConn1 -- Ground3/LConn1
  I/RConn1 -- Conn1/RConn1

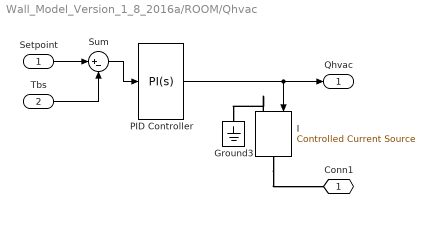
== system Wall_Model_Version_1_8_2016a/ROOM/Qhvac ==
  Setpoint : Inport
  Tbs : Inport  Port=2
  Ground3 : powerlib/Elements/Ground  LConnTagsString=a
  I : powerlib/Electrical Sources/Controlled Current Source  Initialize=on  Source_Type=DC  Amplitude=5000  Phase=0  Frequency=0  Measurements=None
  PID Controller : simulink/Continuous/PID Controller  Controller=PI  TimeDomain=Continuous-time  SampleTime=-1  IntegratorMethod=Backward Euler  FilterMethod=Forward Euler  Form=Parallel  UseFilter=on  ControllerParametersSource=internal  P=226.345300312581  I=107.883047490248  D=-296662.911304383  N=0.0135323447314473  InitialConditionSource=internal  InitialConditionForIntegrator=22  InitialConditionForFilter=0  ExternalReset=none  LimitOutput=on  UpperSaturationLimit=0  LowerSaturationLimit=-15000  LinearizeAsGain=on  AntiWindupMode=none  Kb=1  TrackingMode=off  Kt=1  PParamMin=[]  PParamMax=[]  IParamMin=[]  IParamMax=[]  DParamMin=[]  DParamMax=[]  NParamMin=[]  NParamMax=[]  KbParamMin=[]  KbParamMax=[]  KtParamMin=[]  KtParamMax=[]  POutMin=[]  POutMax=[]  IOutMin=[]  IOutMax=[]  DOutMin=[]  DOutMax=[]  NOutMin=[]  NOutMax=[]  KbOutMin=[]  KbOutMax=[]  KtOutMin=[]  KtOutMax=[]  IntegratorOutMin=[]  IntegratorOutMax=[]  FilterOutMin=[]  FilterOutMax=[]  SumOutMin=[]  SumOutMax=[]  SumI1OutMin=[]  SumI1OutMax=[]  SumI2OutMin=[]  SumI2OutMax=[]  SumI3OutMin=[]  SumI3OutMax=[]  SumDOutMin=[]  SumDOutMax=[]  SaturationOutMin=[]  SaturationOutMax=[]  IntegratorContinuousStateAttributes=''  IntegratorStateMustResolveToSignalObject=off  IntegratorRTWStateStorageClass=Auto  FilterContinuousStateAttributes=''  FilterStateMustResolveToSignalObject=off  FilterRTWStateStorageClass=Auto  DifferentiatorICPrevScaledInput=0  DifferentiatorOutMin=[]  DifferentiatorOutMax=[]
  Sum : Sum  Inputs=|+-
  Conn1 : PMIOPort  Side=Right
  Qhvac : Outport
  wires:
  PID Controller/1 -> I/1, Qhvac/1
  Setpoint/1 -> Sum/1
  Tbs/1 -> Sum/2
  Sum/1 -> PID Controller/1
  connections:
  I/RConn1 -- Conn1/RConn1
  I/LConn1 -- Ground3/LConn1

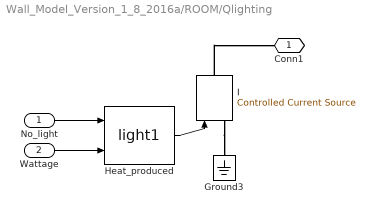
== system Wall_Model_Version_1_8_2016a/ROOM/Qlighting ==
  "No_light " : Inport
  Wattage : Inport  Port=2
  Ground3 : powerlib/Elements/Ground  LConnTagsString=a
  Heat_produced : M-S-Function  FunctionName=light1
  I : powerlib/Electrical Sources/Controlled Current Source  Initialize=on  Source_Type=AC  Amplitude=1  Phase=0  Frequency=0  Measurements=None
  Conn1 : PMIOPort  Side=Right
  wires:
  "No_light "/1 -> Heat_produced/1
  Heat_produced/1 -> I/1
  Wattage/1 -> Heat_produced/2
  connections:
  I/LConn1 -- Ground3/LConn1
  I/RConn1 -- Conn1/RConn1

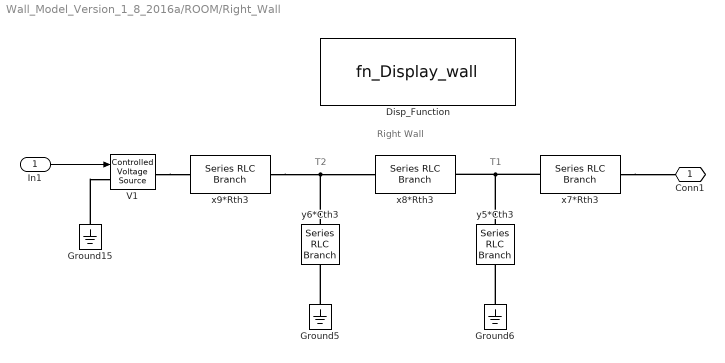
== system Wall_Model_Version_1_8_2016a/ROOM/Right_Wall ==
  note: Right Wall
  note: T2
  note: T1
  In1 : Inport
  Disp_Function : M-S-Function  FunctionName=fn_Display_wall
  Ground15 : powerlib/Elements/Ground  LConnTagsString=a
  Ground5 : powerlib/Elements/Ground  LConnTagsString=a
  Ground6 : powerlib/Elements/Ground  LConnTagsString=a
  V1 : powerlib/Electrical Sources/Controlled Voltage Source  Initialize=on  Source_Type=AC  Amplitude=0  Phase=0  Frequency=0  Measurements=None
  x7*Rth3 : powerlib/Elements/Series RLC Branch  LConnTagsString=__new0  RConnTagsString=__new0  BranchType=R  Resistance=x7*Rth3  Inductance=1e-3  SetiL0=off  InitialCurrent=0  Capacitance=1e-6  Setx0=off  InitialVoltage=0  Measurements=None
  x8*Rth3 : powerlib/Elements/Series RLC Branch  LConnTagsString=__new0  RConnTagsString=__new0  BranchType=R  Resistance=x8*Rth3  Inductance=1e-3  SetiL0=off  InitialCurrent=0  Capacitance=1e-6  Setx0=off  InitialVoltage=0  Measurements=None
  x9*Rth3 : powerlib/Elements/Series RLC Branch  LConnTagsString=__new0  RConnTagsString=__new0  BranchType=R  Resistance=x9*Rth3  Inductance=1e-3  SetiL0=off  InitialCurrent=0  Capacitance=1e-6  Setx0=off  InitialVoltage=0  Measurements=None
  y5*Cth3 : powerlib/Elements/Series RLC Branch  LConnTagsString=__new0  RConnTagsString=__new0  BranchType=C  Resistance=0  Inductance=1e-3  SetiL0=off  InitialCurrent=0  Capacitance=y5*Cth3  Setx0=on  InitialVoltage=T1_initial_right  Measurements=Branch voltage
  y6*Cth3 : powerlib/Elements/Series RLC Branch  LConnTagsString=__new0  RConnTagsString=__new0  BranchType=C  Resistance=0  Inductance=1e-3  SetiL0=off  InitialCurrent=0  Capacitance=y6*Cth3  Setx0=on  InitialVoltage=T2_initial_right  Measurements=Branch voltage
  Conn1 : PMIOPort  Side=Right
  wires:
  In1/1 -> V1/1
  connections:
  x7*Rth3/RConn1 -- Conn1/RConn1
  x7*Rth3/LConn1 -- y5*Cth3/LConn1 -- x8*Rth3/RConn1
  y6*Cth3/LConn1 -- x9*Rth3/RConn1 -- x8*Rth3/LConn1
  Ground15/LConn1 -- V1/LConn1
  Ground5/LConn1 -- y6*Cth3/RConn1
  Ground6/LConn1 -- y5*Cth3/RConn1
  V1/RConn1 -- x9*Rth3/LConn1

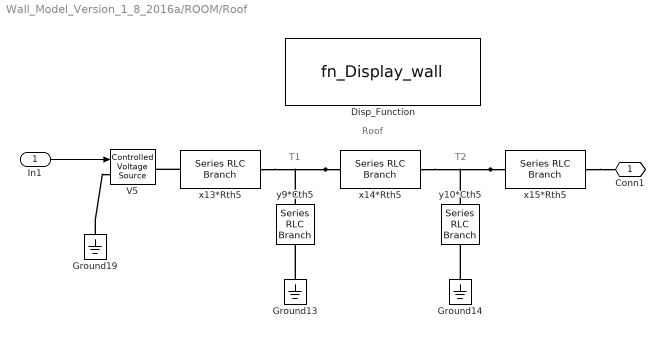
== system Wall_Model_Version_1_8_2016a/ROOM/Roof ==
  note: T1
  note: T2
  note: Roof
  In1 : Inport
  Disp_Function : M-S-Function  FunctionName=fn_Display_wall
  Ground13 : powerlib/Elements/Ground  LConnTagsString=a
  Ground14 : powerlib/Elements/Ground  LConnTagsString=a
  Ground19 : powerlib/Elements/Ground  LConnTagsString=a
  V5 : powerlib/Electrical Sources/Controlled Voltage Source  Initialize=on  Source_Type=AC  Amplitude=0  Phase=0  Frequency=0  Measurements=None
  x13*Rth5 : powerlib/Elements/Series RLC Branch  LConnTagsString=__new0  RConnTagsString=__new0  BranchType=R  Resistance=x13*Rth5  Inductance=1e-3  SetiL0=off  InitialCurrent=0  Capacitance=1e-6  Setx0=off  InitialVoltage=0  Measurements=None
  x14*Rth5 : powerlib/Elements/Series RLC Branch  LConnTagsString=__new0  RConnTagsString=__new0  BranchType=R  Resistance=x14*Rth5  Inductance=1e-3  SetiL0=off  InitialCurrent=0  Capacitance=1e-6  Setx0=off  InitialVoltage=0  Measurements=None
  x15*Rth5 : powerlib/Elements/Series RLC Branch  LConnTagsString=__new0  RConnTagsString=__new0  BranchType=R  Resistance=x15*Rth5  Inductance=1e-3  SetiL0=off  InitialCurrent=0  Capacitance=1e-6  Setx0=off  InitialVoltage=0  Measurements=None
  y10*Cth5 : powerlib/Elements/Series RLC Branch  LConnTagsString=__new0  RConnTagsString=__new0  BranchType=C  Resistance=0  Inductance=1e-3  SetiL0=off  InitialCurrent=0  Capacitance=y10*Cth5  Setx0=on  InitialVoltage=T2_initial_roof  Measurements=Branch voltage
  y9*Cth5 : powerlib/Elements/Series RLC Branch  LConnTagsString=__new0  RConnTagsString=__new0  BranchType=C  Resistance=0  Inductance=1e-3  SetiL0=off  InitialCurrent=0  Capacitance=y9*Cth5  Setx0=on  InitialVoltage=T1_initial_roof  Measurements=Branch voltage
  Conn1 : PMIOPort  Side=Right
  wires:
  In1/1 -> V5/1
  connections:
  Ground14/LConn1 -- y10*Cth5/RConn1
  x15*Rth5/RConn1 -- Conn1/RConn1
  x14*Rth5/LConn1 -- x13*Rth5/RConn1 -- y9*Cth5/LConn1
  x15*Rth5/LConn1 -- x14*Rth5/RConn1 -- y10*Cth5/LConn1
  Ground19/LConn1 -- V5/LConn1
  x13*Rth5/LConn1 -- V5/RConn1
  Ground13/LConn1 -- y9*Cth5/RConn1

== matlab function Wall_Model_Version_1_8_2016a/ROOM/IEQ_INDEX/IAQ_CO2 ==
  data: C input; IAQ_CO2 output
function IAQ_CO2 = fcn(C)
% C in PPM measured 8 hr average
% IAQ
 C_hi = 0; C_lo = 0; I_hi = 0; I_lo = 0;

% Good
if C<400

elseif 400<=C && C<700
    C_hi = 699; C_lo = 400; I_hi = 50; I_lo = 0;
% Moderate
elseif 700<=C && C<1000
    C_hi = 999; C_lo = 700; I_hi = 100; I_lo = 51;
% Unhealthy
elseif 1000<=C && C<1500
    C_hi = 1499; C_lo = 1000; I_hi = 200; I_lo = 101;    
% Very Unhealthy
elseif 1500<=C && C<4500
    C_hi = 4499; C_lo = 1500; I_hi = 300; I_lo = 201;
% Emergency
elseif 4500<=C %&& C<20000
    C_hi = 20000; C_lo = 4500; I_hi = 500; I_lo = 301;    
end

IAQ_CO2 = (((I_hi - I_lo)*(C - C_lo))/(C_hi - C_lo)) + I_lo;

== matlab function Wall_Model_Version_1_8_2016a/ROOM/IEQ_INDEX/IAQ_CO ==
  data: C input; IAQ_CO output
function IAQ_CO = fcn(C)
% C in PPM measured 8 hr average
% IAQ
 C_hi = 0; C_lo = 0; I_hi = 0; I_lo = 0;
 
% Good
if 0<=C && C<5
    C_hi = 4.99; C_lo = 0; I_hi = 50; I_lo = 0;
% Moderate
elseif 5<=C && C<9
    C_hi = 8.99; C_lo = 5; I_hi = 100; I_lo = 51;
% Unhealthy
elseif 9<=C && C<15
    C_hi = 14.99; C_lo = 9; I_hi = 200; I_lo = 101;    
% Very Unhealthy
elseif 15<=C && C<30
    C_hi = 29.99; C_lo = 15; I_hi = 300; I_lo = 201;
% Emergency
elseif 30<=C %&& C<2000
    C_hi = 2000; C_lo = 30; I_hi = 500; I_lo = 301;    
end


IAQ_CO = (((I_hi - I_lo)*(C - C_lo))/(C_hi - C_lo)) + I_lo;

== matlab function Wall_Model_Version_1_8_2016a/ROOM/IEQ_INDEX/IAQ_O3 ==
  data: C input; IAQ_O3 output
function IAQ_O3 = fcn(C)
% C in PPB measured 8 hr average
% IAQ
 C_hi = 0; C_lo = 0; I_hi = 0; I_lo = 0;

% Good
if 0<=C && C<50
    C_hi = 49.9; C_lo = 0; I_hi = 50; I_lo = 0;
% Moderate
elseif 50<=C && C<70
    C_hi = 69.9; C_lo = 50; I_hi = 100; I_lo = 51;
% Unhealthy
elseif 70<=C && C<100
    C_hi = 99.9; C_lo = 70; I_hi = 200; I_lo = 101;    
% Very Unhealthy
elseif 100<=C && C<200
    C_hi = 199.9; C_lo = 100; I_hi = 300; I_lo = 201;
% Emergency
elseif 200<=C %&& C<700
    C_hi = 700; C_lo = 200; I_hi = 500; I_lo = 301;    
end

IAQ_O3 = (((I_hi - I_lo)*(C - C_lo))/(C_hi - C_lo)) + I_lo;

== matlab function Wall_Model_Version_1_8_2016a/ROOM/IEQ_INDEX/IAQ_HCHO ==
  data: C input; IAQ_HCHO output
function IAQ_HCHO = fcn(C)
% C in mg/m3 measured 8 hr average
% IAQ
% reference : https://www.ncbi.nlm.nih.gov/pmc/articles/PMC3175005/
 C_hi = 0; C_lo = 0; I_hi = 0; I_lo = 0;

% Good
if 0<=C && C<0.05
    C_hi = 0.05; C_lo = 0; I_hi = 50; I_lo = 0;
% Moderate
elseif 0.05<=C && C<0.12
    C_hi = 0.119; C_lo = 0.05; I_hi = 100; I_lo = 51;
% Unhealthy
elseif 0.12<=C && C<0.25
    C_hi = 0.249; C_lo =0.12; I_hi = 200; I_lo = 101;    
% Very Unhealthy
elseif 0.25<=C && C<0.6
    C_hi = 0.59; C_lo = 0.25; I_hi = 300; I_lo = 201;
% Emergency
elseif 0.6<=C %&& C<2.5
    C_hi = 2.5; C_lo = 0.6; I_hi = 500; I_lo = 301;    
end

IAQ_HCHO = (((I_hi - I_lo)*(C - C_lo))/(C_hi - C_lo)) + I_lo;

== matlab function Wall_Model_Version_1_8_2016a/ROOM/IEQ_INDEX/IAQ_VOC ==
  data: C input; IAQ_VOC output
function IAQ_VOC = fcn(C)
% C in ppm measured 8 hr average
% IAQ
% reference :THE A DETAILED STUDY OF VOLATILE ORGANIC COMPOUNDS
% OF 5 AIR-CONDITIONED BUILDINGS IN SINGAPORE
% Residential Indoor Air Quality Guideline TOLUENE
 C_hi = 0; C_lo = 0; I_hi = 0; I_lo = 0;

% Good
if 0<=C && C<1.2
    C_hi = 1.19; C_lo = 0; I_hi = 50; I_lo = 0;
% Moderate
elseif 1.2<=C && C<2
    C_hi = 0.119; C_lo = 0.05; I_hi = 100; I_lo = 51;
% Unhealthy
elseif 2<=C && C<3
    C_hi = 2.99; C_lo =2; I_hi = 200; I_lo = 101;    
% Very Unhealthy
elseif 3<=C && C<4
    C_hi = 3.99; C_lo = 3; I_hi = 300; I_lo = 201;
% Emergency
elseif 4<=C %&& C<6
    C_hi = 6; C_lo = 4; I_hi = 500; I_lo = 301;    
end

IAQ_VOC = (((I_hi - I_lo)*(C - C_lo))/(C_hi - C_lo)) + I_lo;

== matlab function Wall_Model_Version_1_8_2016a/ROOM/IEQ_INDEX/IAQ_PM2_5 ==
  data: C input; IAQ_PM2_5 output
function IAQ_PM2_5 = fcn(C)
% C in UG/M3 measured 8 hr average
% IAQ
% reference :THE A DETAILED STUDY OF VOLATILE ORGANIC COMPOUNDS
% OF 5 AIR-CONDITIONED BUILDINGS IN SINGAPORE 
 C_hi = 0; C_lo = 0; I_hi = 0; I_lo = 0;

% Good
if 0<=C && C<10
    C_hi = 9.9; C_lo = 0; I_hi = 50; I_lo = 0;
% Moderate
elseif 10<=C && C<40
    C_hi = 39.9; C_lo = 10; I_hi = 100; I_lo = 51;
% Unhealthy
elseif 40<=C && C<130
    C_hi = 129.9; C_lo = 40; I_hi = 200; I_lo = 101;    
% Very Unhealthy
elseif 130<=C && C<250
    C_hi = 249.9; C_lo = 130; I_hi = 300; I_lo = 201;
% Emergency
elseif 250<=C %&& C<500
    C_hi = 500; C_lo = 250; I_hi = 500; I_lo = 301;    
end

IAQ_PM2_5 = (((I_hi - I_lo)*(C - C_lo))/(C_hi - C_lo)) + I_lo;

== matlab function Wall_Model_Version_1_8_2016a/ROOM/IEQ_INDEX/IAQ_PM10 ==
  data: C input; IAQ_PM10 output
function IAQ_PM10 = fcn(C)
% C in UG/M3 measured 8 hr average
% IAQ
% reference :BCA, SINGAPORE 
 C_hi = 0; C_lo = 0; I_hi = 0; I_lo = 0;

% Good
if 0<=C && C<50
    C_hi = 49.9; C_lo = 0; I_hi = 50; I_lo = 0;
% Moderate
elseif 50<=C && C<150
    C_hi = 149.9; C_lo = 50; I_hi = 100; I_lo = 51;
% Unhealthy
elseif 150<=C && C<350
    C_hi = 349.9; C_lo = 150; I_hi = 200; I_lo = 101;    
% Very Unhealthy
elseif 350<=C && C<425
    C_hi = 424.9; C_lo = 350; I_hi = 300; I_lo = 201;
% Emergency
elseif 425<=C %&& C<600
    C_hi = 600; C_lo = 250; I_hi = 500; I_lo = 301;    
end

IAQ_PM10 = (((I_hi - I_lo)*(C - C_lo))/(C_hi - C_lo)) + I_lo;

== matlab function Wall_Model_Version_1_8_2016a/ROOM/IEQ_INDEX/IEQ_LIGHT ==
  data: C input; IEQ_Light output
function IEQ_Light = fcn(C)
% C in LUX
% IEQ
% reference :https://www.noao.edu/education/QLTkit/ACTIVITY_Documents/Safety/LightLevels_outdoor+indoor.pdf
C_hi = 0; C_lo = 0; I_hi = 0; I_lo = 0;

if 400<=C && C<=600
    C_hi = 600; C_lo = 400; I_hi = 50; I_lo = 0;
% Moderate Comfortable and on darker side
elseif 200<=C && C <400
    C_hi = 399; C_lo = 200; I_hi = 75; I_lo = 51;
% Moderate Comfortable and on brighter side
elseif 600<C && C <1000
    C_hi = 999; C_lo = 601; I_hi = 75; I_lo = 51;     
% UnComfortable and Too Bright
elseif C >= 1000 && C<5000
    C_hi =5000; C_lo = 1000; I_hi = 100; I_lo = 76;
% UnComfortable and Too Dark
elseif C >= 0 && C<200
    C_hi =199; C_lo = 0; I_hi = 100; I_lo = 76;    
end

IEQ_Light = (((I_hi - I_lo)*(C - C_lo))/(C_hi - C_lo)) + I_lo;

== matlab function Wall_Model_Version_1_8_2016a/ROOM/IEQ_INDEX/PMV ==
  data: CLO input; PMV_index output; MET input; TA input; TR input; VEL input; RH input; PPD output
%Computer program (BASIC) for calculation of
% Predicted Mean Vote (PMV) and Predicted Percentage of Dissatisfaction (PPD)
% in accordance with ISO 7730
% INPUT “ Clothing (clo)” ; CLO
% INPUT “ Metabolic rate (met)” ; MET
% INPUT “ External work, normally around 0 (met)” ; WME
% INPUT “ Air Temperature (DEG K )” ; TA 
% INPUT “ Mean radiant temperature (DEG K )” ; TR
% INPUT “ Relative air velocity (m/s)” : VEL
% INPUT “ Relative humidity ( % )” ; RH


% CLO = 1;  % clothing
% MET = 1.1;  % metabolic rate
% WME = 0  ;  % external work
% TA  = 25.7+273 ;  % air temperature
% TR  = 25.7+273 ;  % mean radiant temperature
% VEL = 0.1;  % relative air velocity
% RH  = 15 ;  % relative humidity

function [PMV_index,PPD] = PMV(CLO,MET,TA,TR,VEL,RH)
TA  = TA - 273;
TR  =TR -273;
FNPS= exp(16.6536-4030.183/(TA + 235)); % saturated vapor pressure KPa
PA  = RH * 10 * FNPS; % water vapor pressure, Pa
ICL = .155 * CLO; % thermal insulation of the clothing in m2K/W
M   = MET * 58.15; % metabolic rate in W/m2
W   = 0; % external work in W/m2
MW  = M - W;  % internal heat production in the human body
% clothing area factor
if (ICL < .078) 
    FCL = 1 + 1.29 * ICL; 
else
    FCL = 1.05+0.645*ICL;
end
HCF = 12.1*sqrt(VEL) ; % heat transf. coefficient by forced convection
TAA = TA + 273; % air temperature in Kelvin
TRA = TR + 273; % mean radiant temperature in Kelvin

%%  CACULATE SURFACE TEMPERATURE OF CLOTHING BY ITERATION - - - - - - - - - - - - - - - -
TCLA = TAA + (35.5-TA) / (3.5*(6.45*ICL+.1)); % first guess for surface temperature of clothing
P1 = ICL * FCL; % calculation term
P2 = P1 * 3.96; % calculation term
P3 = P1 * 100; %calculation term
P4 = P1 * TAA; %calculation term
P5 = 308.7 -.028 * MW +P2 * (TRA/100) ^ 4; % calculation term
XN = TCLA / 100;
XF = XN;
EPS = .00015;% stop criteria in iteration

%% heat transf. coeff. by natural convection
XF = (XF+XN) / 2; 
HCN=2.38*abs(100*XF-TAA)^.25;
if (HCF>HCN)
    HC=HCF; 
else
    HC=HCN;
end
XN=(P5+P4*HC-P2*XF^4) / (100+P3*HC);
TCL = 100*XN - 273; 
while(abs(XN-XF) > EPS)
    XF = (XF+XN) / 2; % heat transf. coeff. by natural convection
    HCN=2.38*abs(100*XF-TAA)^.25;
    if (HCF>HCN)
        HC=HCF; 
    else
        HC=HCN;
    end
    XN=(P5+P4*HC-P2*XF^4) / (100+P3*HC);
    TCL=100*XN-273; % surface temperature of the clothing

end

%%  HEAT LOSS COMPONENTS
HL1 = 3.05*.001*(5733-6.99*MW-PA); % heat loss diff. through skin
% heat loss by sweating (comfort)
if (MW > 58.15) 
    HL2 = .42 * (MW - 58.15);
else
    HL2 =1;
end
% latent respiration heat loss
HL3 = 1.7 * .00001 * M * (5867-PA);
% dry respiration heat loss
HL4 = .0014 * M * (34-TA);
% heat loss by radiation
HL5 = 3.96*FCL*(XN^4-(TRA/100)^4);
% heat loss by convection
HL6 = FCL * HC * (TCL-TA);


%% CALCULATE PMV AND PPD 
% thermal sensation trans. Coeff.
TS = .303 * exp(-.036*M) + 0.028;
% predicted mean vote
PMV_index = TS * (MW-HL1-HL2-HL3-HL4-HL5-HL6);
% predicted percentage dissat.
PPD=100-95*exp(-.03353*PMV_index^4-.2179*PMV_index^2);
end
